simulink model "model"  (R2021a)
settings: Solver=FixedStepAuto  StartTime=0.0  StopTime=24*3600  FixedStep=60  RelTol=1e-3
model workspace (MAT data in the model file):
  x = Simulink.Bus
  x.Alignment = -1
  x.PreserveElementDimensions = 0
  x.DataScope = 'Auto'
undefined symbols (not defined in the file): DiscIntNeverNeededParam
libraries: simulink x5, fuzblock x2, mlepLibrary x1, embmathops x1
settings Model: PauseTimes=21000  Creator=E592090  LastModifiedBy=migue
settings SolverCC: DecoupledContinuousIntegration=on
settings DataIOCC: SaveOutput=off  DSMLogging=off
settings DebuggingCC: ReadBeforeWriteMsg=DisableAll  WriteAfterWriteMsg=DisableAll  WriteAfterReadMsg=DisableAll  MultiTaskDSMMsg=none  SFMachineParentedDataDiag=warning  ArithmeticOperatorsInVariantConditions=warning
settings ModelReferenceCC: UpdateModelReferenceTargets=IfOutOfDate
settings SFSimCC: SFSimEcho=off  SimUseLocalCustomCode=off  CustomCodeUndefinedFunction=UseInterfaceOnly
settings RTWCC: RTWUseLocalCustomCode=off

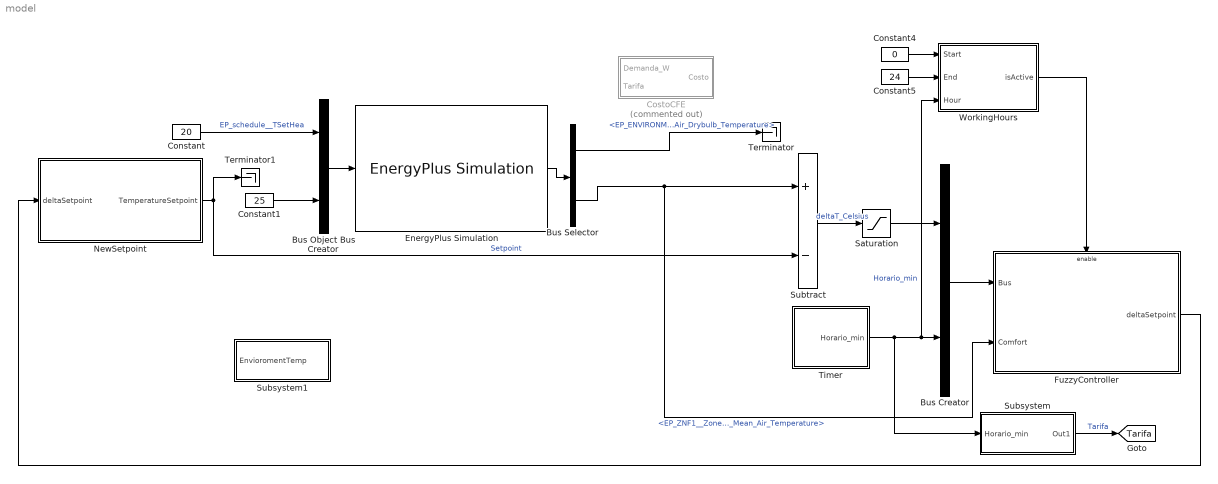
== system model ==
  Bus Creator : BusCreator  Inputs=2
  Bus Selector : BusSelector  OutputSignals=EP_ENVIRONMENT__Site_Outdoor_Air_Drybulb_Temperature,EP_ZNF1__Zone_Mean_Air_Temperature
  Bus Object Bus Creator : BusCreator  Inputs=2  mask(Bus Object Bus Creator){busType=Select a Bus object...}
      mask prompts: busType "Bus Type"
      mask help:
      | Provides users the cabability to painlessly, instantly customize bus creators of output data type 'Bus:' by selecting the bus object type from a drop down menu dynamically populated by bus objects in the workspace.
      |
      | After pressing the "Apply Selection" button signal lines into the creator are populated and named with the elements in the chosen bus saving the user from having to recall and fill out signal line names.
      |
      | NOTE that when copying a Bus Object Bus Creator from your locked Library the link to the Library is automatically broken. This saves the user from having to Unlock Links To Library (From the Library menu.), Disable Link and finally Break Link (Both from the Model menu.) for every placed instance of the block.
      settings: AttributesFormatString=%<OutDataTypeStr>  CopyFcn=busObjectBusCreator_clbk(gcb,'CopyFcn');
      mask TypeOptions busType: Select a Bus object... | Bus: epInbus | Bus: epOutbus
      mask Callback busType: busObjectBusCreator_clbk(gcb,'popup');
      mask DialogControl applyMOCBSelection Prompt: Apply Selection
      mask DialogControl applyMOCBSelection Callback: busObjectBusCreator_clbk(gcb,'button');
  Constant : Constant  Value=20
  Constant1 : Constant  Value=25
  Constant4 : Constant  Value=0
  Constant5 : Constant  Value=24
  CostoCFE : Subsystem  Commented=on
  EnergyPlus Simulation : mlepLibrary/EnergyPlus Simulation  Priority=1  idfFile=C:\git\boreas\EnergyPlus\examples\legacy_example\SmOffPSZ.idf  epwFile=C:\git\boreas\Simulation\Weather\USA_IL_Chicago-OHare.Intl.AP.725300_TMY3.epw  inputBusName=epInbus  outputBusName=epOutbus  useDataDictionary=off  dataDictionaryName=EnergyPlusSimulation.sldd
      settings: SourceProductName=EnergyPlus co-simulation toolbox
  FuzzyController : Subsystem  TreatAsAtomicUnit=on
  NewSetpoint : Subsystem
  Saturation : Saturate  UpperLimit=10  LowerLimit=0
  Subsystem : Subsystem
  Subsystem1 : Subsystem
  Subtract : Sum  Inputs=+-
  Terminator : Terminator
  Terminator1 : Terminator
  Timer : Subsystem
  WorkingHours : Subsystem
  tag scope: Tarifa=global
  wires:
  Bus Object Bus Creator/1 -> EnergyPlus Simulation/1
  Constant/1 -> Bus Object Bus Creator/1  "EP_schedule__TSetHea"
  EnergyPlus Simulation/1 -> Bus Selector/1
  Bus Selector/2 -> FuzzyController/2(Comfort), Subtract/1  "<EP_ZNF1__Zone_Mean_Air_Temperature>"
  Subtract/1 -> Saturation/1  "deltaT_Celsius"
  Bus Creator/1 -> FuzzyController/1(Bus)
  Timer/1(Horario_min) -> Bus Creator/2, WorkingHours/3(Hour), Subsystem/1(Horario_min)  "Horario_min"
  NewSetpoint/1(TemperatureSetpoint) -> Terminator1/1, Subtract/2  "Setpoint"
  FuzzyController/1(deltaSetpoint) -> NewSetpoint/1(deltaSetpoint)
  Constant4/1 -> WorkingHours/1(Start)
  Constant5/1 -> WorkingHours/2(End)
  WorkingHours/1(isActive) -> FuzzyController/Enable
  Subsystem/1(Out1) -> [Tarifa]  "Tarifa"
  Bus Selector/1 -> Terminator/1  "<EP_ENVIRONMENT__Site_Outdoor_Air_Drybulb_Temperature>"
  Saturation/1 -> Bus Creator/1
  Constant1/1 -> Bus Object Bus Creator/2

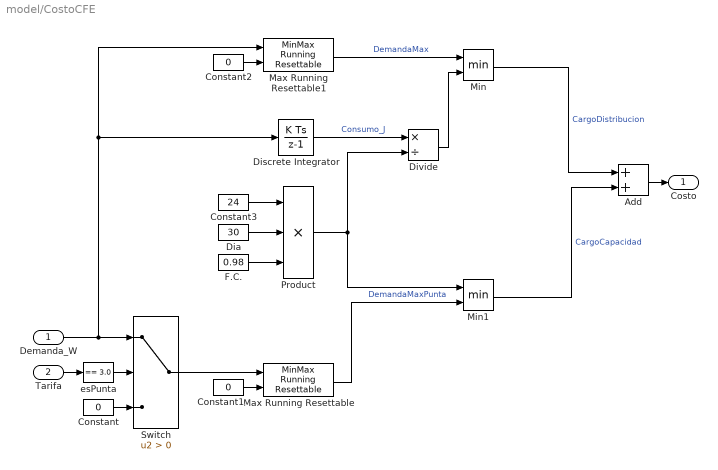
== system model/CostoCFE ==
  Demanda_W : Inport
  Tarifa : Inport  Port=2
  Add : Sum
  Constant : Constant  Value=0
  Constant1 : Constant  Value=0
  Constant2 : Constant  Value=0
  Constant3 : Constant  Value=24
  Dia : Constant  Value=30
  Discrete Integrator : DiscreteIntegrator  SampleTime=-1  ICPrevOutput=DiscIntNeverNeededParam  ICPrevScaledInput=DiscIntNeverNeededParam
  Divide : Product  Inputs=*/
  F.C. : Constant  Value=0.98
  Max Running Resettable : simulink/Math Operations/MinMax Running Resettable  Function=max  vinit=0.0
  Max Running Resettable1 : simulink/Math Operations/MinMax Running Resettable  Function=max  vinit=0.0
  Min : MinMax  Inputs=2
  Min1 : MinMax  Inputs=2
  Product : Product  Inputs=3
  Switch : Switch  Criteria=u2 > Threshold
  esPunta : simulink/Logic and Bit Operations/Compare To Constant  relop===  const=3.0  OutDataTypeStr=boolean
  Costo : Outport
  wires:
  Tarifa/1 -> esPunta/1
  Demanda_W/1 -> Max Running Resettable1/1, Discrete Integrator/1, Switch/1
  esPunta/1 -> Switch/2
  Constant/1 -> Switch/3
  Switch/1 -> Max Running Resettable/1
  Constant1/1 -> Max Running Resettable/2
  Constant2/1 -> Max Running Resettable1/2
  Dia/1 -> Product/2
  Constant3/1 -> Product/1
  F.C./1 -> Product/3
  Discrete Integrator/1 -> Divide/1  "Consumo_J"
  Max Running Resettable1/1 -> Min/1  "DemandaMax"
  Divide/1 -> Min/2
  Product/1 -> Min1/1, Divide/2
  Max Running Resettable/1 -> Min1/2  "DemandaMaxPunta"
  Min/1 -> Add/1  "CargoDistribucion"
  Min1/1 -> Add/2  "CargoCapacidad"
  Add/1 -> Costo/1

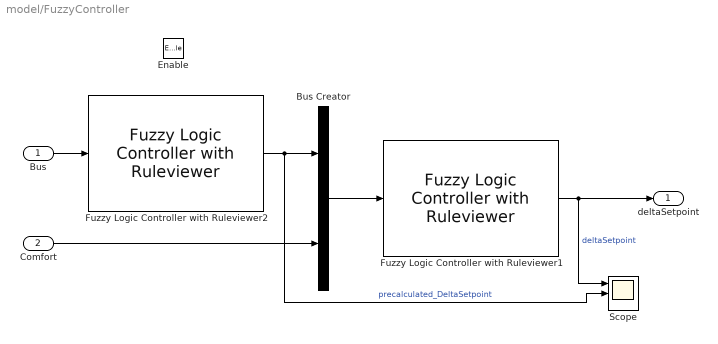
== system model/FuzzyController ==
  Bus : Inport
  Comfort : Inport  Port=2
  Enable : EnablePort
  Bus Creator : BusCreator  Inputs=2
  Fuzzy Logic Controller with Ruleviewer1 : fuzblock/Fuzzy Logic  Controller  with Ruleviewer  fismatrix=fis2  Ts=60*30
  Fuzzy Logic Controller with Ruleviewer2 : fuzblock/Fuzzy Logic  Controller  with Ruleviewer  fismatrix=fis1  Ts=60*30
  Scope : Scope  NumInputPorts=3
  deltaSetpoint : Outport
  wires:
  Comfort/1 -> Bus Creator/2
  Bus Creator/1 -> Fuzzy Logic Controller with Ruleviewer1/1
  Fuzzy Logic Controller with Ruleviewer1/1 -> Scope/1, deltaSetpoint/1  "deltaSetpoint"
  Fuzzy Logic Controller with Ruleviewer2/1 -> Scope/2, Bus Creator/1  "precalculated_DeltaSetpoint"
  Bus/1 -> Fuzzy Logic Controller with Ruleviewer2/1

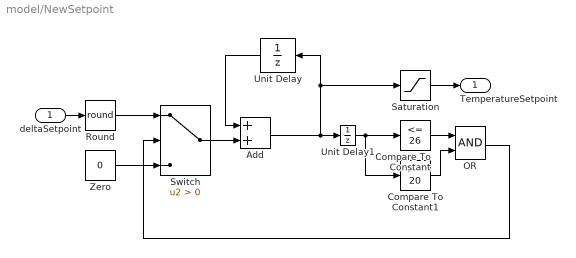
== system model/NewSetpoint ==
  deltaSetpoint : Inport
  Add : Sum
  Compare To Constant : simulink/Logic and Bit Operations/Compare To Constant  relop=<=  const=26  OutDataTypeStr=boolean
  Compare To Constant1 : simulink/Logic and Bit Operations/Compare To Constant  relop=>=  const=20  OutDataTypeStr=boolean
  OR : Logic  AllPortsSameDT=off  OutDataTypeStr=boolean
  Round : Rounding  Operator=round
  Saturation : Saturate  UpperLimit=26  LowerLimit=20
  Switch : Switch  Criteria=u2 > Threshold
  Unit Delay : UnitDelay  InitialCondition=25  SampleTime=-1  HasFrameUpgradeWarning=on
  Unit Delay1 : UnitDelay  SampleTime=-1  HasFrameUpgradeWarning=on
  Zero : Constant  Value=0  OutDataTypeStr=Inherit: Inherit via back propagation
  TemperatureSetpoint : Outport
  wires:
  Unit Delay/1 -> Add/1
  Zero/1 -> Switch/3
  Switch/1 -> Add/2
  Compare To Constant/1 -> OR/1
  Compare To Constant1/1 -> OR/2
  OR/1 -> Switch/2
  Saturation/1 -> TemperatureSetpoint/1
  Add/1 -> Unit Delay1/1, Saturation/1, Unit Delay/1
  Unit Delay1/1 -> Compare To Constant1/1, Compare To Constant/1
  deltaSetpoint/1 -> Round/1
  Round/1 -> Switch/1

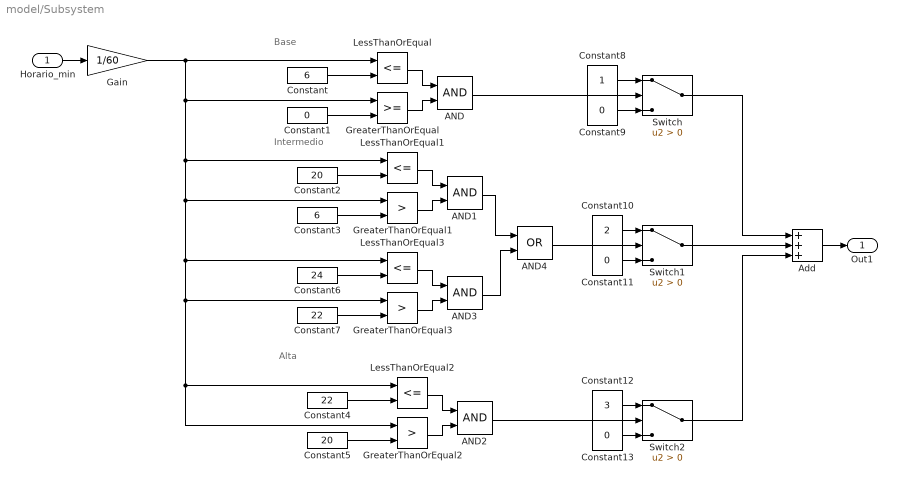
== system model/Subsystem ==
  note: Alta
  note: Intermedio
  note: Base
  Horario_min : Inport
  AND{,1..3} (4 alike) : Logic  AllPortsSameDT=off  OutDataTypeStr=boolean
  AND4 : Logic  Operator=OR  AllPortsSameDT=off  OutDataTypeStr=boolean
  Add : Sum  Inputs=+++
  Constant : Constant  Value=6
  Constant{1,9,11,13} (4 alike) : Constant  Value=0
  Constant10 : Constant  Value=2
  Constant12 : Constant  Value=3
  Constant2 : Constant  Value=20
  Constant3 : Constant  Value=6
  Constant4 : Constant  Value=22
  Constant5 : Constant  Value=20
  Constant6 : Constant  Value=24
  Constant7 : Constant  Value=22
  Constant8 : Constant
  Gain : Gain  Gain=1/60
  GreaterThanOrEqual : RelationalOperator  OutDataTypeStr=boolean  RndMeth=Simplest
  GreaterThanOrEqual1 : RelationalOperator  Operator=>  OutDataTypeStr=boolean  RndMeth=Simplest
  GreaterThanOrEqual2 : RelationalOperator  Operator=>  OutDataTypeStr=boolean  RndMeth=Simplest
  GreaterThanOrEqual3 : RelationalOperator  Operator=>  OutDataTypeStr=boolean  RndMeth=Simplest
  LessThanOrEqual{,1..3} (4 alike) : RelationalOperator  Operator=<=  OutDataTypeStr=boolean  RndMeth=Simplest
  Switch : Switch  Criteria=u2 > Threshold
  Switch1 : Switch  Criteria=u2 > Threshold
  Switch2 : Switch  Criteria=u2 > Threshold
  Out1 : Outport
  wires:
  Horario_min/1 -> Gain/1
  Constant/1 -> LessThanOrEqual/2
  Constant1/1 -> GreaterThanOrEqual/2
  LessThanOrEqual/1 -> AND/1
  GreaterThanOrEqual/1 -> AND/2
  Constant2/1 -> LessThanOrEqual1/2
  GreaterThanOrEqual1/1 -> AND1/2
  Constant3/1 -> GreaterThanOrEqual1/2
  LessThanOrEqual1/1 -> AND1/1
  Constant4/1 -> LessThanOrEqual2/2
  GreaterThanOrEqual2/1 -> AND2/2
  Constant5/1 -> GreaterThanOrEqual2/2
  LessThanOrEqual2/1 -> AND2/1
  GreaterThanOrEqual3/1 -> AND3/2
  LessThanOrEqual3/1 -> AND3/1
  Constant6/1 -> LessThanOrEqual3/2
  Constant7/1 -> GreaterThanOrEqual3/2
  AND1/1 -> AND4/1
  AND3/1 -> AND4/2
  Gain/1 -> GreaterThanOrEqual1/1, LessThanOrEqual3/1, GreaterThanOrEqual3/1, LessThanOrEqual2/1, GreaterThanOrEqual2/1, LessThanOrEqual1/1, GreaterThanOrEqual/1, LessThanOrEqual/1
  AND/1 -> Switch/2
  AND4/1 -> Switch1/2
  AND2/1 -> Switch2/2
  Constant8/1 -> Switch/1
  Constant9/1 -> Switch/3
  Constant10/1 -> Switch1/1
  Constant11/1 -> Switch1/3
  Constant12/1 -> Switch2/1
  Constant13/1 -> Switch2/3
  Switch1/1 -> Add/2
  Switch/1 -> Add/1
  Switch2/1 -> Add/3
  Add/1 -> Out1/1

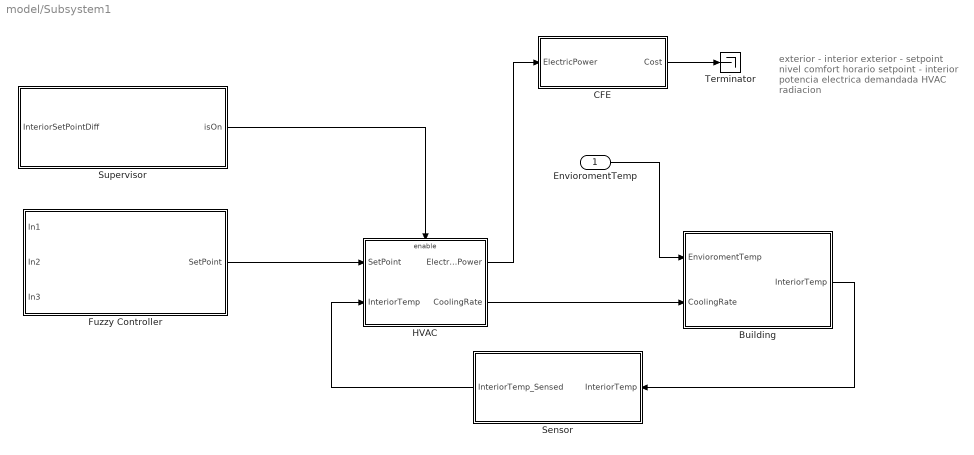
== system model/Subsystem1 ==
  note: exterior - interior
      | exterior - setpoint
      | nivel comfort
      | horario
      | setpoint - interior
      | potencia electrica demandada HVAC
      | radiacion
  EnvioromentTemp : Inport
  Building : Subsystem
  CFE : Subsystem
  Fuzzy Controller : Subsystem  TreatAsAtomicUnit=on
  HVAC : Subsystem
  Sensor : Subsystem
  Supervisor : Subsystem
  Terminator : Terminator
  wires:
  HVAC/2(CoolingRate) -> Building/2(CoolingRate)
  Fuzzy Controller/1(SetPoint) -> HVAC/1(SetPoint)
  Supervisor/1(isOn) -> HVAC/Enable
  Building/1(InteriorTemp) -> Sensor/1(InteriorTemp)
  Sensor/1(InteriorTemp_Sensed) -> HVAC/2(InteriorTemp)
  HVAC/1(ElectricPower) -> CFE/1(ElectricPower)
  EnvioromentTemp/1 -> Building/1(EnvioromentTemp)
  CFE/1(Cost) -> Terminator/1

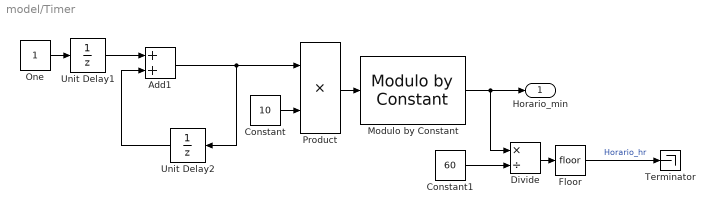
== system model/Timer ==
  Add1 : Sum
  Constant : Constant  Value=10
  Constant1 : Constant  Value=60
  Divide : Product  Inputs=*/
  Floor : Rounding
  Modulo by Constant : embmathops/Modulo by Constant  Denominator=1440  SimulateUsing=Code generation
      settings: SourceProductBaseCode=SL
  One : Constant  OutDataTypeStr=Inherit: Inherit via back propagation
  Product : Product
  Terminator : Terminator
  Unit Delay1 : UnitDelay  SampleTime=-1  HasFrameUpgradeWarning=on
  Unit Delay2 : UnitDelay  SampleTime=-1  HasFrameUpgradeWarning=on
  Horario_min : Outport
  wires:
  One/1 -> Unit Delay1/1
  Unit Delay1/1 -> Add1/1
  Add1/1 -> Unit Delay2/1, Product/1
  Unit Delay2/1 -> Add1/2
  Constant/1 -> Product/2
  Product/1 -> Modulo by Constant/1
  Modulo by Constant/1 -> Divide/1, Horario_min/1
  Constant1/1 -> Divide/2
  Divide/1 -> Floor/1
  Floor/1 -> Terminator/1  "Horario_hr"

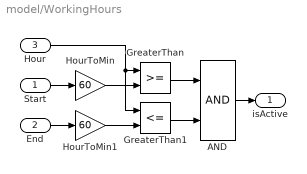
== system model/WorkingHours ==
  Start : Inport
  End : Inport  Port=2
  Hour : Inport  Port=3
  AND : Logic  AllPortsSameDT=off  OutDataTypeStr=boolean
  GreaterThan : RelationalOperator  OutDataTypeStr=boolean  RndMeth=Simplest
  GreaterThan1 : RelationalOperator  Operator=<=  OutDataTypeStr=boolean  RndMeth=Simplest
  HourToMin : Gain  Gain=60
  HourToMin1 : Gain  Gain=60
  isActive : Outport
  wires:
  GreaterThan/1 -> AND/1
  End/1 -> HourToMin1/1
  Start/1 -> HourToMin/1
  HourToMin1/1 -> GreaterThan1/2
  Hour/1 -> GreaterThan1/1, GreaterThan/1
  GreaterThan1/1 -> AND/2
  HourToMin/1 -> GreaterThan/2
  AND/1 -> isActive/1

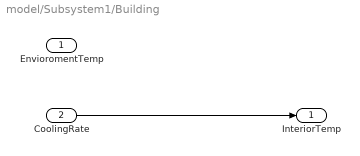
== system model/Subsystem1/Building ==
  EnvioromentTemp : Inport
  CoolingRate : Inport  Port=2
  InteriorTemp : Outport
  wires:
  CoolingRate/1 -> InteriorTemp/1

== system model/Subsystem1/CFE ==
  ElectricPower : Inport
  Cost : Outport
  wires:
  ElectricPower/1 -> Cost/1

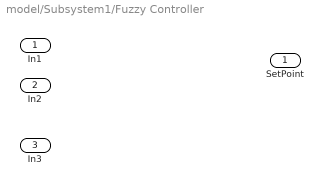
== system model/Subsystem1/Fuzzy Controller ==
  In1 : Inport
  In2 : Inport  Port=2
  In3 : Inport  Port=3
  SetPoint : Outport

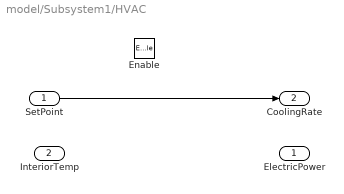
== system model/Subsystem1/HVAC ==
  SetPoint : Inport
  InteriorTemp : Inport  Port=2
  Enable : EnablePort
  ElectricPower : Outport
  CoolingRate : Outport  Port=2
  wires:
  SetPoint/1 -> CoolingRate/1

== system model/Subsystem1/Sensor ==
  InteriorTemp : Inport
  InteriorTemp_Sensed : Outport
  wires:
  InteriorTemp/1 -> InteriorTemp_Sensed/1

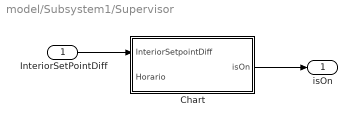
== system model/Subsystem1/Supervisor ==
  InteriorSetPointDiff : Inport
  Chart : Stateflow chart  TreatAsAtomicUnit=on
  isOn : Outport
  wires:
  InteriorSetPointDiff/1 -> Chart/1(InteriorSetpointDiff)
  Chart/1(isOn) -> isOn/1

== stateflow chart model/Subsystem1/Supervisor/Chart ==
  state Prendido
    en:
    isOn = true;
  state Apagado
    en:
    isOn = false;
  (default) -> Prendido
  Prendido -> Apagado : [InteriorSetpointDiff <= 1 || (Horario == 3 && InteriorSetpointDiff < 3) ]
  Apagado -> Prendido : [(InteriorSetpointDiff >= 3 && Horario ~= 3) || InteriorSetpointDiff > 4 ]
  data: InteriorSetpointDiff input; isOn output; Horario input
